simulink model "BPiKU_BAT"  (R2018b)
settings: Solver=ode23t  StartTime=0.0  StopTime=4  RelTol=1e-6
undefined symbols (not defined in the file): Cdc, i_kt_int, i_kt_p, LdM, Lout, Rd, RdM, sigbuilder_block, u_k_int, u_k_p
libraries: powerlib x29, simulink x5, powerlib_meascontrol x3
settings Model: SimulationMode=accelerator  Creator=K2  LastModifiedBy=K2

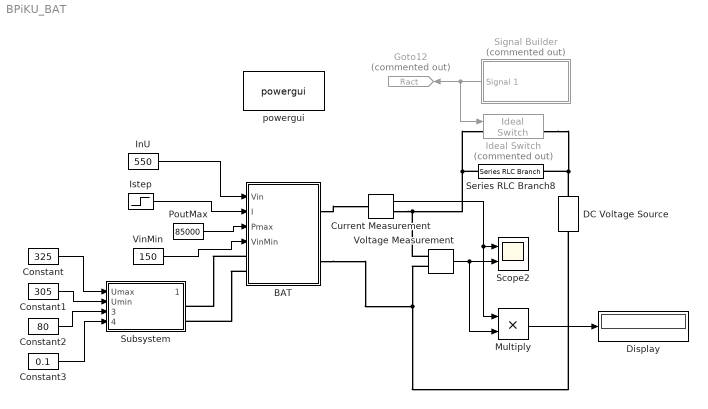
== system BPiKU_BAT ==
  BAT : Subsystem
  Constant : Constant  Value=325
  Constant1 : Constant  Value=305
  Constant2 : Constant  Value=80
  Constant3 : Constant  Value=0.1
  Current Measurement : powerlib/Measurements/Current Measurement  PhasorSimulation=off  OutputType=Complex  PSBequivalent=0
  DC Voltage Source : powerlib/Electrical Sources/DC Voltage Source  Amplitude=0  Measurements=None
  Display : Display
      settings: Format=bank
  Goto12 : Goto  Commented=on  GotoTag=Ract  TagVisibility=global
  Ideal Switch : powerlib/Power Electronics/Ideal Switch  Commented=on  Ron=550*550/85000  Lon=0  IC=0  Rs=1e5  Cs=inf  Measurements=on
  InU : Constant  Value=550
  Istep : Step  Time=0.01  After=85000/320  SampleTime=1/freq/2
  Multiply : Product
  PoutMax : Constant  Value=85000  SampleTime=0
  Scope2 : Scope  NumInputPorts=2
  Series RLC Branch8 : powerlib/Elements/Series RLC Branch  LConnTagsString=__new0  RConnTagsString=__new0  BranchType=R  Resistance=550*550/85000  Inductance=10e-6  SetiL0=off  InitialCurrent=0  Capacitance=1000e-6  Setx0=off  InitialVoltage=0  Measurements=None
  Signal Builder : Subsystem  Tag=STV Subsys  Commented=on  LoadFcn=sigbuilder_block('load');  StartFcn=sigbuilder_block('start');  StopFcn=sigbuilder_block('stop');  ClipboardFcn=sigbuilder_block('clipboard');  mask(Sigbuilder block){tuvar=[0:10]}
      mask help: Simulink:masks:SigbuilderBlock_MD
      mask init:
      | if ~strcmp(get_param(bdroot(gcbh),'SimulationStatus'),'stopped') tuvar = sigbuilder_block('maskInit'); end
      settings: CopyFcn=sigbuilder_block('copy');  DeleteFcn=sigbuilder_block('delete');  ModelCloseFcn=sigbuilder_block('modelClose');  PreSaveFcn=sigbuilder_block('preSave');  PauseFcn=sigbuilder_block('pause');  ContinueFcn=sigbuilder_block('continue');  NameChangeFcn=sigbuilder_block('namechange');  OpenFcn=sigbuilder_block('open',[193.5 84.75 550.5 399.75 ]);  CloseFcn=sigbuilder_block('close');
      mask Display: plot(0, 0, 100, 100,[2, 2, 32, 32, 2], [68, 8, 8, 68, 68],[32, 2], [38, 38], [32, 19, 2],[53, 60, 44], [32, 17, 17, 2],[16, 16, 31, 31]);txt = getActiveGroup(gcbh);text(2, 100, txt,'verticalAlignment', 'top');
  Subsystem : Subsystem
  VinMin : Constant  Value=150  SampleTime=0
  Voltage Measurement : powerlib/Measurements/Voltage Measurement  PhasorSimulation=off  OutputType=Complex  PSBequivalent=0
  powergui : powerlib/powergui  Priority=1  SimulationMode=Discrete  SampleTime=1e-6  frequency=60  Iterations=50  frequencyindice=0  Pbase=100e6  ErrMax=1e-4  UnitsV=kV  UnitsW=MW  buscounter=0  FunctionMessages=off  echomessages=off  EnableUseOfTLC=off  CurrentSourceSwitches=off  DisableSnubberDevices=off  DisableRonSwitches=off  DisableVfSwitches=off  DisplayEquations=off  SolverType=Backward Euler  Interpol=off  ExternalGateDelay=off  methode=off  Ts=100  x0status=blocks  SPID=off  SwTol=0  HookPort=off  RestoreLinks=warning  ResistiveCurrentMeasurement=off  Frange=[0:2:500]  Ylog=off  Xlog=on  ShowGrid=off  save=off  variable=ZData  structure=0  ZoomFFT=off  StartTime=0.0  cycles=1  DisplayStyle=1  fundamental=60  FreqAxis=off  MaxFrequency=1000  frequencyindicesteady=1  RmsSteady=1  display=off
  wires:
  Signal Builder/1(Signal 1) -> Ideal Switch/1, Goto12/1
  InU/1 -> BAT/1(Vin)
  Istep/1 -> BAT/2(I)
  PoutMax/1 -> BAT/3(Pmax)
  Current Measurement/1 -> Multiply/1, Scope2/1
  Voltage Measurement/1 -> Multiply/2, Scope2/2
  Multiply/1 -> Display/1
  Constant/1 -> Subsystem/1(Umax)
  Constant1/1 -> Subsystem/2(Umin)
  Constant2/1 -> Subsystem/3(InitSOC%)
  Constant3/1 -> Subsystem/4(CapMaxAh)
  VinMin/1 -> BAT/4(VinMin)
  connections:
  DC Voltage Source/RConn1 -- Ideal Switch/RConn1 -- Series RLC Branch8/RConn1
  Series RLC Branch8/LConn1 -- Voltage Measurement/LConn1 -- Current Measurement/RConn1 -- Ideal Switch/LConn1
  Voltage Measurement/LConn2 -- BAT/RConn2 -- DC Voltage Source/LConn1
  BAT/RConn1 -- Current Measurement/LConn1
  BAT/LConn1 -- Subsystem/RConn1
  BAT/LConn2 -- Subsystem/RConn2

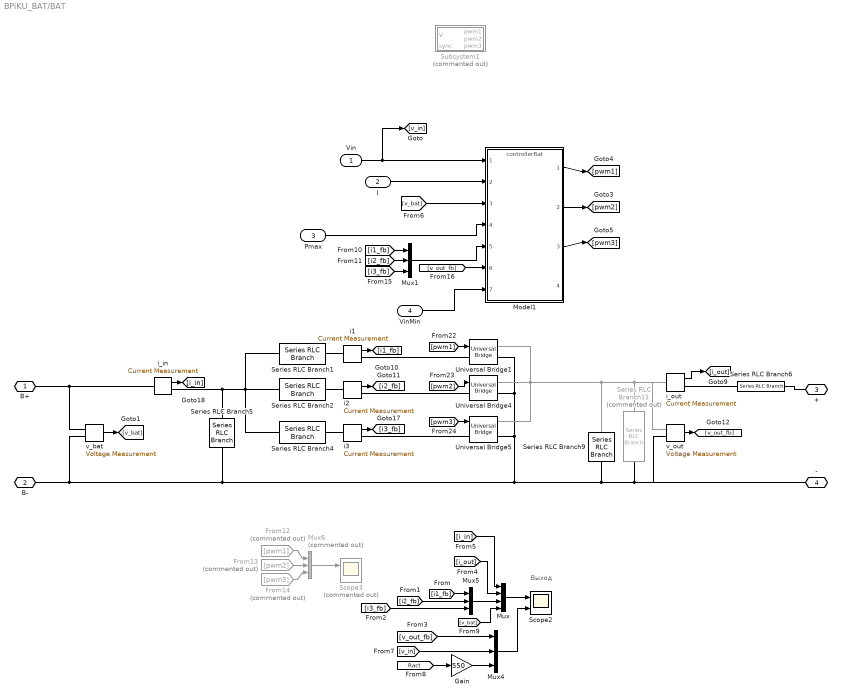
== system BPiKU_BAT/BAT ==
  note: Выход
  Vin : Inport
  I : Inport  Port=2
  Pmax : Inport  Port=3
  VinMin : Inport  Port=4
  From12 : From  Commented=on  GotoTag=pwm1
  From13 : From  Commented=on  GotoTag=pwm2
  From14 : From  Commented=on  GotoTag=pwm3
  Gain : Gain  Gain=550
  Model1 : ModelReference  ModelNameDialog=controllerBat.slx  SimulationMode=Normal  ModelReferenceVersion=1.6
  Mux : Mux
  Mux1 : Mux  Inputs=3
  Mux4 : Mux  Inputs=3
  Mux5 : Mux  Inputs=3
  Mux6 : Mux  Commented=on  Inputs=3
  Scope2 : Scope  NumInputPorts=2
  Scope3 : Scope  Commented=on  NumInputPorts=2
  Series RLC Branch1 : powerlib/Elements/Series RLC Branch  LConnTagsString=__new0  RConnTagsString=__new0  BranchType=RL  Resistance=RdM(1)  Inductance=LdM(1)  SetiL0=off  InitialCurrent=0  Capacitance=100e-6  Setx0=off  InitialVoltage=0  Measurements=None
  Series RLC Branch11 : powerlib/Elements/Series RLC Branch  Commented=on  LConnTagsString=__new0  RConnTagsString=__new0  BranchType=Open circuit  Resistance=2000  Inductance=50e-6  SetiL0=off  InitialCurrent=0  Capacitance=100e-6  Setx0=off  InitialVoltage=0  Measurements=None
  Series RLC Branch2 : powerlib/Elements/Series RLC Branch  LConnTagsString=__new0  RConnTagsString=__new0  BranchType=RL  Resistance=RdM(2)  Inductance=LdM(2)  SetiL0=off  InitialCurrent=0  Capacitance=100e-6  Setx0=off  InitialVoltage=0  Measurements=None
  Series RLC Branch4 : powerlib/Elements/Series RLC Branch  LConnTagsString=__new0  RConnTagsString=__new0  BranchType=RL  Resistance=RdM(3)  Inductance=LdM(3)  SetiL0=off  InitialCurrent=0  Capacitance=100e-6  Setx0=off  InitialVoltage=0  Measurements=None
  Series RLC Branch5 : powerlib/Elements/Series RLC Branch  LConnTagsString=__new0  RConnTagsString=__new0  BranchType=C  Resistance=0.0001  Inductance=50e-6  SetiL0=off  InitialCurrent=0  Capacitance=8000e-6  Setx0=on  InitialVoltage=300  Measurements=None
  Series RLC Branch6 : powerlib/Elements/Series RLC Branch  LConnTagsString=__new0  RConnTagsString=__new0  BranchType=RL  Resistance=Rd  Inductance=Lout  SetiL0=off  InitialCurrent=0  Capacitance=1e-6  Setx0=off  InitialVoltage=0  Measurements=None
  Series RLC Branch9 : powerlib/Elements/Series RLC Branch  LConnTagsString=__new0  RConnTagsString=__new0  BranchType=C  Resistance=0.0001  Inductance=50e-6  SetiL0=off  InitialCurrent=0  Capacitance=Cdc  Setx0=on  InitialVoltage=550  Measurements=None
  Subsystem1 : Subsystem  Commented=on
  Universal Bridge1 : powerlib/Power Electronics/Universal Bridge  Arms=1  SnubberResistance=1e5  SnubberCapacitance=inf  Device=MOSFET / Diodes  Ron=1e-3  Lon=0  ForwardVoltages="[  2  2  ]"  ForwardVoltage=0  GTOparameters=[ 10e-6 , 20e-6 ]  IGBTparameters=[ 1e-6 , 2e-6 ]  Measurements=None  Measurements_2=None  converterType=Rectifier
  Universal Bridge4 : powerlib/Power Electronics/Universal Bridge  Arms=1  SnubberResistance=1e5  SnubberCapacitance=inf  Device=MOSFET / Diodes  Ron=1e-3  Lon=0  ForwardVoltages="[  2  2  ]"  ForwardVoltage=0  GTOparameters=[ 10e-6 , 20e-6 ]  IGBTparameters=[ 1e-6 , 2e-6 ]  Measurements=None  Measurements_2=None  converterType=Rectifier
  Universal Bridge5 : powerlib/Power Electronics/Universal Bridge  Arms=1  SnubberResistance=1e5  SnubberCapacitance=inf  Device=MOSFET / Diodes  Ron=1e-3  Lon=0  ForwardVoltages="[  2  2  ]"  ForwardVoltage=0  GTOparameters=[ 10e-6 , 20e-6 ]  IGBTparameters=[ 1e-6 , 2e-6 ]  Measurements=None  Measurements_2=None  converterType=Rectifier
  i1 : powerlib/Measurements/Current Measurement  PhasorSimulation=off  OutputType=Complex  PSBequivalent=0
  i2 : powerlib/Measurements/Current Measurement  PhasorSimulation=off  OutputType=Complex  PSBequivalent=0
  i3 : powerlib/Measurements/Current Measurement  PhasorSimulation=off  OutputType=Complex  PSBequivalent=0
  i_in : powerlib/Measurements/Current Measurement  PhasorSimulation=off  OutputType=Complex  PSBequivalent=0
  i_out : powerlib/Measurements/Current Measurement  PhasorSimulation=off  OutputType=Complex  PSBequivalent=0
  v_bat : powerlib/Measurements/Voltage Measurement  PhasorSimulation=off  OutputType=Complex  PSBequivalent=0
  v_out : powerlib/Measurements/Voltage Measurement  PhasorSimulation=off  OutputType=Complex  PSBequivalent=0
  B+ : PMIOPort  Side=Left
  B- : PMIOPort  Port=2  Side=Left
  + : PMIOPort  Port=3  Side=Right
  - : PMIOPort  Port=4  Side=Right
  wires:
  From14/1 -> Mux6/3
  From12/1 -> Mux6/1
  [v_in] -> Mux4/2
  Mux5/1 -> Mux/3
  [v_out_fb] -> Mux4/1
  Mux/1 -> Scope2/1
  [i_in] -> Mux/1
  [i_out] -> Mux/2
  [i1_fb] -> Mux5/1
  From13/1 -> Mux6/2
  Mux6/1 -> Scope3/1
  [i2_fb] -> Mux5/2
  Mux4/1 -> Scope2/2
  [i3_fb] -> Mux5/3
  i3/1 -> [i3_fb]
  i1/1 -> [i1_fb]
  i2/1 -> [i2_fb]
  i_in/1 -> [i_in]
  [pwm3] -> Universal Bridge5/1
  [pwm2] -> Universal Bridge4/1
  [pwm1] -> Universal Bridge1/1
  i_out/1 -> [i_out]
  v_out/1 -> [v_out_fb]
  Model1/2 -> [pwm2]
  Model1/1 -> [pwm1]
  Vin/1 -> Model1/1, [v_in]
  Model1/3 -> [pwm3]
  I/1 -> Model1/2
  v_bat/1 -> [v_bat]
  [v_bat] -> Model1/3
  [Ract] -> Gain/1
  Gain/1 -> Mux4/3
  Pmax/1 -> Model1/4
  [v_bat] -> Mux/4
  [i2_fb] -> Mux1/2
  [i3_fb] -> Mux1/3
  [i1_fb] -> Mux1/1
  Mux1/1 -> Model1/5
  [v_out_fb] -> Model1/6
  VinMin/1 -> Model1/7
  connections:
  i_in/RConn1 -- Series RLC Branch5/LConn1 -- Series RLC Branch4/LConn1 -- Series RLC Branch2/LConn1 -- Series RLC Branch1/LConn1
  i1/LConn1 -- Series RLC Branch1/RConn1
  i3/LConn1 -- Series RLC Branch4/RConn1
  i2/RConn1 -- Universal Bridge4/LConn1
  i1/RConn1 -- Universal Bridge1/LConn1
  i2/LConn1 -- Series RLC Branch2/RConn1
  Universal Bridge5/LConn1 -- i3/RConn1
  Series RLC Branch6/RConn1 -- i_out/RConn1
  Universal Bridge5/RConn2 -- Series RLC Branch9/RConn1 -- Series RLC Branch11/RConn1 -- v_out/LConn2 -- -/RConn1 -- Series RLC Branch5/RConn1 -- v_bat/LConn2 -- B-/RConn1 -- Universal Bridge1/RConn2 -- Universal Bridge4/RConn2
  B+/RConn1 -- v_bat/LConn1 -- i_in/LConn1
  +/RConn1 -- Series RLC Branch6/LConn1
  Series RLC Branch11/LConn1 -- v_out/LConn1 -- i_out/LConn1 -- Universal Bridge5/RConn1 -- Universal Bridge1/RConn1 -- Universal Bridge4/RConn1 -- Series RLC Branch9/LConn1

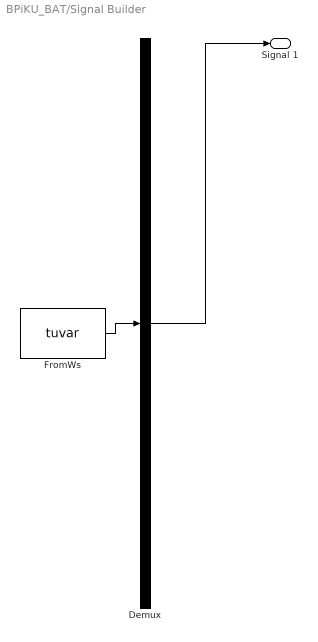
== system BPiKU_BAT/Signal Builder ==
  Demux : Demux  Tag=STV Demux  Outputs=1
  FromWs : FromWorkspace  Tag=STV FromWs  VariableName=tuvar  SampleTime=0
      SigBuilderData=|
      | common.afterFinalStr = 'Extrapolate'
      | common.sampleTime = 0
      | dataSet.timeRange = [0 10]
      | dataSet.name = 'Group 1'
      | sbobj.Groups.Name = 'Group 1'
      | sbobj.Groups.Signals.Name = 'Signal 1'
      | sbobj.Groups.Signals.XData = [0 0.02 0.51 0.51 1.5 1.5 1.88 1.88 2 2 2.07 2.07 2.15 2.15 2.24 2.24 3.58 3.58 6 10]
      | sbobj.Groups.Signals.YData = [0 0 0 1 1 0 0 1 1 0 0 1 1 0 0 1 1 0 0 0]
  Signal 1 : Outport  Tag=STV Outport
  wires:
  Demux/1 -> Signal 1/1
  FromWs/1 -> Demux/1

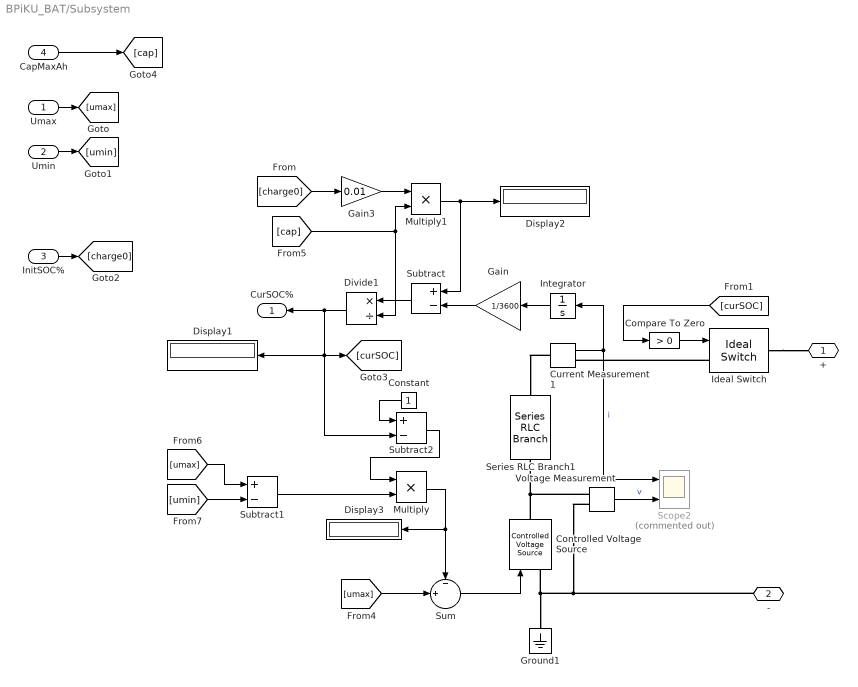
== system BPiKU_BAT/Subsystem ==
  Umax : Inport
  Umin : Inport  Port=2
  InitSOC% : Inport  Port=3
  CapMaxAh : Inport  Port=4
  Compare To Zero : simulink/Logic and Bit Operations/Compare To Zero  relop=>  OutDataTypeStr=boolean
  Constant : Constant
  Controlled Voltage Source : powerlib/Electrical Sources/Controlled Voltage Source  Initialize=on  Source_Type=AC  Amplitude=0  Phase=0  Frequency=0  Measurements=None
  Current Measurement1 : powerlib/Measurements/Current Measurement  PhasorSimulation=off  OutputType=Complex  PSBequivalent=0
  Display1 : Display
  Display2 : Display
  Display3 : Display
  Divide1 : Product  Inputs=*/
  Gain : Gain  Gain=1/3600
  Gain3 : Gain  Gain=0.01
  Ground1 : powerlib/Elements/Ground  LConnTagsString=a
  Ideal Switch : powerlib/Power Electronics/Ideal Switch  Ron=0.001  Lon=0  IC=0  Rs=1e5  Cs=inf  Measurements=off
  Integrator : Integrator
  Multiply : Product
  Multiply1 : Product
  Scope2 : Scope  Commented=on  NumInputPorts=2
  Series RLC Branch1 : powerlib/Elements/Series RLC Branch  LConnTagsString=__new0  RConnTagsString=__new0  BranchType=R  Resistance=0.01  Inductance=10e-6  SetiL0=off  InitialCurrent=0  Capacitance=1000e-6  Setx0=off  InitialVoltage=0  Measurements=None
  Subtract : Sum  Inputs=+-
  Subtract1 : Sum  Inputs=+-
  Subtract2 : Sum  Inputs=+-
  Sum : Sum  Inputs=-|+||
  Voltage Measurement : powerlib/Measurements/Voltage Measurement  PhasorSimulation=off  OutputType=Complex  PSBequivalent=0
  + : PMIOPort  Side=Right
  - : PMIOPort  Port=2  Side=Right
  CurSOC% : Outport
  wires:
  [umax] -> Sum/2
  Sum/1 -> Controlled Voltage Source/1
  Integrator/1 -> Gain/1
  Voltage Measurement/1 -> Scope2/2  "v"
  Current Measurement1/1 -> Scope2/1, Integrator/1  "i"
  Divide1/1 -> [curSOC], Subtract2/2, Display1/1, CurSOC%/1
  Umax/1 -> [umax]
  Umin/1 -> [umin]
  InitSOC%/1 -> [charge0]
  CapMaxAh/1 -> [cap]
  [charge0] -> Gain3/1
  Gain3/1 -> Multiply1/1
  [cap] -> Divide1/2, Multiply1/2
  Multiply1/1 -> Subtract/1, Display2/1
  Gain/1 -> Subtract/2
  Subtract/1 -> Divide1/1
  [umax] -> Subtract1/1
  [umin] -> Subtract1/2
  Subtract1/1 -> Multiply/2
  Multiply/1 -> Display3/1, Sum/1
  Constant/1 -> Subtract2/1
  Subtract2/1 -> Multiply/1
  [curSOC] -> Compare To Zero/1
  Compare To Zero/1 -> Ideal Switch/1
  connections:
  -/RConn1 -- Voltage Measurement/LConn2 -- Ground1/LConn1 -- Controlled Voltage Source/LConn1
  Current Measurement1/LConn1 -- Series RLC Branch1/LConn1
  Controlled Voltage Source/RConn1 -- Voltage Measurement/LConn1 -- Series RLC Branch1/RConn1
  Ideal Switch/LConn1 -- Current Measurement1/RConn1
  Ideal Switch/RConn1 -- +/RConn1

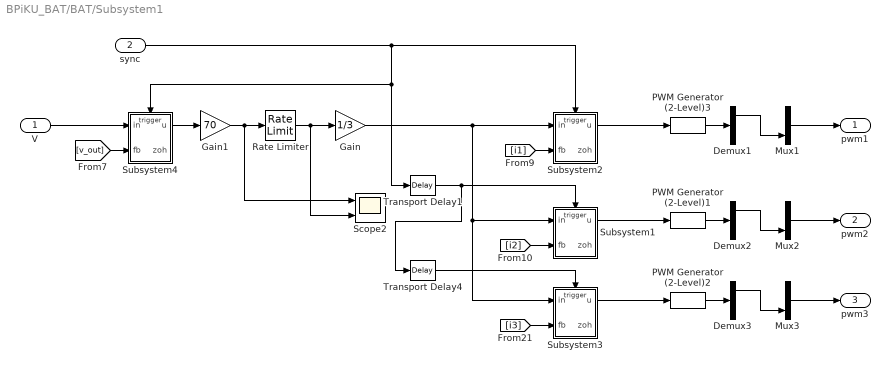
== system BPiKU_BAT/BAT/Subsystem1 ==
  V : Inport
  sync : Inport  Port=2
  Demux1 : Demux  Outputs=2
  Demux2 : Demux  Outputs=2
  Demux3 : Demux  Outputs=2
  Gain : Gain  Gain=1/3
  Gain1 : Gain  Gain=70
  Mux1 : Mux  Inputs=2
  Mux2 : Mux  Inputs=2
  Mux3 : Mux  Inputs=2
  PWM Generator (2-Level)1 : powerlib_meascontrol/Pulse & Signal Generators/PWM Generator (2-Level)  ModulatorType=Single-phase half-bridge (2 pulses)  ModulatorMode=Unsynchronized  Fc=freq  Pc=120  nF=1  MinMax="[0.001  1 ]"  SamplingTechnique=Natural  ModulatingSignals=off  m=0.8  Freq=60  Phase=0  Ts=0  ShowCarrierOutport=off
      settings: SourceProductName=Simscape Power Systems
  PWM Generator (2-Level)2 : powerlib_meascontrol/Pulse & Signal Generators/PWM Generator (2-Level)  ModulatorType=Single-phase half-bridge (2 pulses)  ModulatorMode=Unsynchronized  Fc=freq  Pc=-120  nF=1  MinMax="[0.001  1 ]"  SamplingTechnique=Natural  ModulatingSignals=off  m=0.8  Freq=60  Phase=0  Ts=0  ShowCarrierOutport=off
      settings: SourceProductName=Simscape Power Systems
  PWM Generator (2-Level)3 : powerlib_meascontrol/Pulse & Signal Generators/PWM Generator (2-Level)  ModulatorType=Single-phase half-bridge (2 pulses)  ModulatorMode=Unsynchronized  Fc=freq  Pc=0  nF=1  MinMax="[0.001  1 ]"  SamplingTechnique=Natural  ModulatingSignals=off  m=0.8  Freq=60  Phase=0  Ts=0  ShowCarrierOutport=off
      settings: SourceProductName=Simscape Power Systems
  Rate Limiter : RateLimiter  RisingSlewLimit=15  FallingSlewLimit=-15  SampleTimeMode=inherited
  Scope2 : Scope  NumInputPorts=2
  Subsystem1 : Subsystem
  Subsystem2 : Subsystem
  Subsystem3 : Subsystem
  Subsystem4 : Subsystem
  Transport Delay1 : TransportDelay  DelayTime=1/freq/2/3
  Transport Delay4 : TransportDelay  DelayTime=1/freq/2/3
  pwm1 : Outport
  pwm2 : Outport  Port=2
  pwm3 : Outport  Port=3
  wires:
  [i2] -> Subsystem1/2(fb)
  [i3] -> Subsystem3/2(fb)
  sync/1 -> Subsystem4/Trigger, Transport Delay1/1, Subsystem2/Trigger
  Transport Delay1/1 -> Subsystem1/Trigger, Transport Delay4/1
  Transport Delay4/1 -> Subsystem3/Trigger
  Mux1/1 -> pwm1/1
  Subsystem2/1(u) -> PWM Generator (2-Level)3/1
  PWM Generator (2-Level)3/1 -> Demux1/1
  Demux1/1 -> Mux1/2
  V/1 -> Subsystem4/1(in)
  [i1] -> Subsystem2/2(fb)
  Gain/1 -> Subsystem3/1(in), Subsystem1/1(in), Subsystem2/1(in)
  PWM Generator (2-Level)2/1 -> Demux3/1
  PWM Generator (2-Level)1/1 -> Demux2/1
  Mux2/1 -> pwm2/1
  [v_out] -> Subsystem4/2(fb)
  Subsystem3/1(u) -> PWM Generator (2-Level)2/1
  Demux2/1 -> Mux2/2
  Demux3/1 -> Mux3/2
  Subsystem1/1(u) -> PWM Generator (2-Level)1/1
  Subsystem4/1(u) -> Gain1/1
  Mux3/1 -> pwm3/1
  Rate Limiter/1 -> Scope2/2, Gain/1
  Gain1/1 -> Scope2/1, Rate Limiter/1

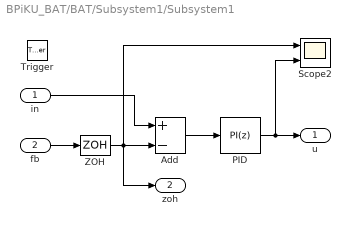
== system BPiKU_BAT/BAT/Subsystem1/Subsystem1 ==
  in : Inport
  fb : Inport  Port=2
  Trigger : TriggerPort  VariantControl=Variant  PortDimensions=1
  Add : Sum  Inputs=+-
  PID : simulink/Continuous/PID Controller  Controller=PI  Form=Parallel  TimeDomain=Discrete-time  SampleTime=-1  IntegratorMethod=Forward Euler  FilterMethod=Forward Euler  ControllerParametersSource=internal  P=i_kt_p  I=i_kt_int  D=0  UseFilter=on  N=100  TunerSelectOption=Transfer Function Based (PID Tuner App)  InitialConditionSource=internal  InitialConditionForIntegrator=0  InitialConditionForFilter=0  DifferentiatorICPrevScaledInput=0  ExternalReset=none  TrackingMode=off  Kt=1  LimitOutput=on  UpperSaturationLimit=1  LowerSaturationLimit=0  LinearizeAsGain=on  AntiWindupMode=none  Kb=1  POutMin=[]  POutMax=[]  IOutMin=[]  IOutMax=[]  DOutMin=[]  DOutMax=[]  NOutMin=[]  NOutMax=[]  SumOutMin=[]  SumOutMax=[]  SaturationOutMin=[]  SaturationOutMax=[]  PParamMin=[]  PParamMax=[]  IParamMin=[]  IParamMax=[]  DParamMin=[]  DParamMax=[]  NParamMin=[]  NParamMax=[]  KbParamMin=[]  KbParamMax=[]  KtParamMin=[]  KtParamMax=[]  KbOutMin=[]  KbOutMax=[]  KtOutMin=[]  KtOutMax=[]  IntegratorOutMin=[]  IntegratorOutMax=[]  FilterOutMin=[]  FilterOutMax=[]  SumI1OutMin=[]  SumI1OutMax=[]  SumI2OutMin=[]  SumI2OutMax=[]  SumI3OutMin=[]  SumI3OutMax=[]  SumI4OutMin=[]  SumI4OutMax=[]  SumDOutMin=[]  SumDOutMax=[]  DifferentiatorOutMin=[]  DifferentiatorOutMax=[]  FilterDiffOutCoefMin=[]  FilterDiffOutCoefMax=[]  ReciprocalOutMin=[]  ReciprocalOutMax=[]  SumDenOutMin=[]  SumDenOutMax=[]  SumNumOutMin=[]  SumNumOutMax=[]  DivideOutMin=[]  DivideOutMax=[]  IntegratorContinuousStateAttributes=''  IntegratorStateMustResolveToSignalObject=off  IntegratorRTWStateStorageClass=Auto  FilterContinuousStateAttributes=''  FilterStateMustResolveToSignalObject=off  FilterRTWStateStorageClass=Auto  ParallelPVariant=InternalParameters  IdealPVariant=Disabled  IVariant=InternalParameters  DVariant=Disabled  IntegratorVariant=Discrete  SatVariant=Enabled  AWVariant=Passthrough  PCopyVariant=Disabled  TRVariant=Disabled  FdbkBlocksVariant=Forward  IdealPFdbkVariant=Disabled  SatFdbkVariant=Disabled  DerivativeFilterVariant=Disabled  NVariant=Disabled  NCopyVariant=Disabled_SignalSpec  FilterICVariant=Disabled  IntegratorICVariant=InternalICs  ExternalResetVariant=Disabled  TRSumVariant=Passthrough  SumFdbkVariant=Disabled  SumVariant=Sum_PI
  Scope2 : Scope  NumInputPorts=2
  ZOH : ZeroOrderHold  SampleTime=-1
  u : Outport
  zoh : Outport  Port=2
  wires:
  fb/1 -> ZOH/1
  in/1 -> Add/1
  Add/1 -> PID/1
  PID/1 -> Scope2/2, u/1
  ZOH/1 -> Scope2/1, zoh/1, Add/2

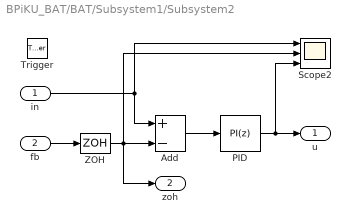
== system BPiKU_BAT/BAT/Subsystem1/Subsystem2 ==
  in : Inport
  fb : Inport  Port=2
  Trigger : TriggerPort  VariantControl=Variant  PortDimensions=1
  Add : Sum  Inputs=+-
  PID : simulink/Continuous/PID Controller  Controller=PI  Form=Parallel  TimeDomain=Discrete-time  SampleTime=-1  IntegratorMethod=Forward Euler  FilterMethod=Forward Euler  ControllerParametersSource=internal  P=i_kt_p  I=i_kt_int  D=0  UseFilter=on  N=100  TunerSelectOption=Transfer Function Based (PID Tuner App)  InitialConditionSource=internal  InitialConditionForIntegrator=0  InitialConditionForFilter=0  DifferentiatorICPrevScaledInput=0  ExternalReset=none  TrackingMode=off  Kt=1  LimitOutput=on  UpperSaturationLimit=1  LowerSaturationLimit=0  LinearizeAsGain=on  AntiWindupMode=none  Kb=1  POutMin=[]  POutMax=[]  IOutMin=[]  IOutMax=[]  DOutMin=[]  DOutMax=[]  NOutMin=[]  NOutMax=[]  SumOutMin=[]  SumOutMax=[]  SaturationOutMin=[]  SaturationOutMax=[]  PParamMin=[]  PParamMax=[]  IParamMin=[]  IParamMax=[]  DParamMin=[]  DParamMax=[]  NParamMin=[]  NParamMax=[]  KbParamMin=[]  KbParamMax=[]  KtParamMin=[]  KtParamMax=[]  KbOutMin=[]  KbOutMax=[]  KtOutMin=[]  KtOutMax=[]  IntegratorOutMin=[]  IntegratorOutMax=[]  FilterOutMin=[]  FilterOutMax=[]  SumI1OutMin=[]  SumI1OutMax=[]  SumI2OutMin=[]  SumI2OutMax=[]  SumI3OutMin=[]  SumI3OutMax=[]  SumI4OutMin=[]  SumI4OutMax=[]  SumDOutMin=[]  SumDOutMax=[]  DifferentiatorOutMin=[]  DifferentiatorOutMax=[]  FilterDiffOutCoefMin=[]  FilterDiffOutCoefMax=[]  ReciprocalOutMin=[]  ReciprocalOutMax=[]  SumDenOutMin=[]  SumDenOutMax=[]  SumNumOutMin=[]  SumNumOutMax=[]  DivideOutMin=[]  DivideOutMax=[]  IntegratorContinuousStateAttributes=''  IntegratorStateMustResolveToSignalObject=off  IntegratorRTWStateStorageClass=Auto  FilterContinuousStateAttributes=''  FilterStateMustResolveToSignalObject=off  FilterRTWStateStorageClass=Auto  ParallelPVariant=InternalParameters  IdealPVariant=Disabled  IVariant=InternalParameters  DVariant=Disabled  IntegratorVariant=Discrete  SatVariant=Enabled  AWVariant=Passthrough  PCopyVariant=Disabled  TRVariant=Disabled  FdbkBlocksVariant=Forward  IdealPFdbkVariant=Disabled  SatFdbkVariant=Disabled  DerivativeFilterVariant=Disabled  NVariant=Disabled  NCopyVariant=Disabled_SignalSpec  FilterICVariant=Disabled  IntegratorICVariant=InternalICs  ExternalResetVariant=Disabled  TRSumVariant=Passthrough  SumFdbkVariant=Disabled  SumVariant=Sum_PI
  Scope2 : Scope  NumInputPorts=3
  ZOH : ZeroOrderHold  SampleTime=-1
  u : Outport
  zoh : Outport  Port=2
  wires:
  fb/1 -> ZOH/1
  in/1 -> Scope2/1, Add/1
  Add/1 -> PID/1
  PID/1 -> Scope2/3, u/1
  ZOH/1 -> Scope2/2, zoh/1, Add/2

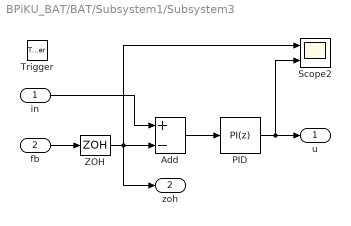
== system BPiKU_BAT/BAT/Subsystem1/Subsystem3 ==
  in : Inport
  fb : Inport  Port=2
  Trigger : TriggerPort  VariantControl=Variant  PortDimensions=1
  Add : Sum  Inputs=+-
  PID : simulink/Continuous/PID Controller  Controller=PI  Form=Parallel  TimeDomain=Discrete-time  SampleTime=-1  IntegratorMethod=Forward Euler  FilterMethod=Forward Euler  ControllerParametersSource=internal  P=i_kt_p  I=i_kt_int  D=0  UseFilter=on  N=100  TunerSelectOption=Transfer Function Based (PID Tuner App)  InitialConditionSource=internal  InitialConditionForIntegrator=0  InitialConditionForFilter=0  DifferentiatorICPrevScaledInput=0  ExternalReset=none  TrackingMode=off  Kt=1  LimitOutput=on  UpperSaturationLimit=1  LowerSaturationLimit=0  LinearizeAsGain=on  AntiWindupMode=none  Kb=1  POutMin=[]  POutMax=[]  IOutMin=[]  IOutMax=[]  DOutMin=[]  DOutMax=[]  NOutMin=[]  NOutMax=[]  SumOutMin=[]  SumOutMax=[]  SaturationOutMin=[]  SaturationOutMax=[]  PParamMin=[]  PParamMax=[]  IParamMin=[]  IParamMax=[]  DParamMin=[]  DParamMax=[]  NParamMin=[]  NParamMax=[]  KbParamMin=[]  KbParamMax=[]  KtParamMin=[]  KtParamMax=[]  KbOutMin=[]  KbOutMax=[]  KtOutMin=[]  KtOutMax=[]  IntegratorOutMin=[]  IntegratorOutMax=[]  FilterOutMin=[]  FilterOutMax=[]  SumI1OutMin=[]  SumI1OutMax=[]  SumI2OutMin=[]  SumI2OutMax=[]  SumI3OutMin=[]  SumI3OutMax=[]  SumI4OutMin=[]  SumI4OutMax=[]  SumDOutMin=[]  SumDOutMax=[]  DifferentiatorOutMin=[]  DifferentiatorOutMax=[]  FilterDiffOutCoefMin=[]  FilterDiffOutCoefMax=[]  ReciprocalOutMin=[]  ReciprocalOutMax=[]  SumDenOutMin=[]  SumDenOutMax=[]  SumNumOutMin=[]  SumNumOutMax=[]  DivideOutMin=[]  DivideOutMax=[]  IntegratorContinuousStateAttributes=''  IntegratorStateMustResolveToSignalObject=off  IntegratorRTWStateStorageClass=Auto  FilterContinuousStateAttributes=''  FilterStateMustResolveToSignalObject=off  FilterRTWStateStorageClass=Auto  ParallelPVariant=InternalParameters  IdealPVariant=Disabled  IVariant=InternalParameters  DVariant=Disabled  IntegratorVariant=Discrete  SatVariant=Enabled  AWVariant=Passthrough  PCopyVariant=Disabled  TRVariant=Disabled  FdbkBlocksVariant=Forward  IdealPFdbkVariant=Disabled  SatFdbkVariant=Disabled  DerivativeFilterVariant=Disabled  NVariant=Disabled  NCopyVariant=Disabled_SignalSpec  FilterICVariant=Disabled  IntegratorICVariant=InternalICs  ExternalResetVariant=Disabled  TRSumVariant=Passthrough  SumFdbkVariant=Disabled  SumVariant=Sum_PI
  Scope2 : Scope  NumInputPorts=2
  ZOH : ZeroOrderHold  SampleTime=-1
  u : Outport
  zoh : Outport  Port=2
  wires:
  fb/1 -> ZOH/1
  in/1 -> Add/1
  Add/1 -> PID/1
  PID/1 -> Scope2/2, u/1
  ZOH/1 -> Scope2/1, zoh/1, Add/2

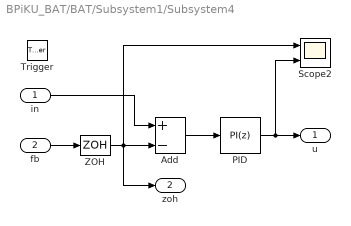
== system BPiKU_BAT/BAT/Subsystem1/Subsystem4 ==
  in : Inport
  fb : Inport  Port=2
  Trigger : TriggerPort  VariantControl=Variant  PortDimensions=1
  Add : Sum  Inputs=+-
  PID : simulink/Continuous/PID Controller  Controller=PI  Form=Parallel  TimeDomain=Discrete-time  SampleTime=-1  IntegratorMethod=Forward Euler  FilterMethod=Forward Euler  ControllerParametersSource=internal  P=u_k_p  I=u_k_int  D=0  UseFilter=on  N=100  TunerSelectOption=Transfer Function Based (PID Tuner App)  InitialConditionSource=internal  InitialConditionForIntegrator=0  InitialConditionForFilter=0  DifferentiatorICPrevScaledInput=0  ExternalReset=none  TrackingMode=off  Kt=1  LimitOutput=on  UpperSaturationLimit=1  LowerSaturationLimit=0  LinearizeAsGain=on  AntiWindupMode=none  Kb=1  POutMin=[]  POutMax=[]  IOutMin=[]  IOutMax=[]  DOutMin=[]  DOutMax=[]  NOutMin=[]  NOutMax=[]  SumOutMin=[]  SumOutMax=[]  SaturationOutMin=[]  SaturationOutMax=[]  PParamMin=[]  PParamMax=[]  IParamMin=[]  IParamMax=[]  DParamMin=[]  DParamMax=[]  NParamMin=[]  NParamMax=[]  KbParamMin=[]  KbParamMax=[]  KtParamMin=[]  KtParamMax=[]  KbOutMin=[]  KbOutMax=[]  KtOutMin=[]  KtOutMax=[]  IntegratorOutMin=[]  IntegratorOutMax=[]  FilterOutMin=[]  FilterOutMax=[]  SumI1OutMin=[]  SumI1OutMax=[]  SumI2OutMin=[]  SumI2OutMax=[]  SumI3OutMin=[]  SumI3OutMax=[]  SumI4OutMin=[]  SumI4OutMax=[]  SumDOutMin=[]  SumDOutMax=[]  DifferentiatorOutMin=[]  DifferentiatorOutMax=[]  FilterDiffOutCoefMin=[]  FilterDiffOutCoefMax=[]  ReciprocalOutMin=[]  ReciprocalOutMax=[]  SumDenOutMin=[]  SumDenOutMax=[]  SumNumOutMin=[]  SumNumOutMax=[]  DivideOutMin=[]  DivideOutMax=[]  IntegratorContinuousStateAttributes=''  IntegratorStateMustResolveToSignalObject=off  IntegratorRTWStateStorageClass=Auto  FilterContinuousStateAttributes=''  FilterStateMustResolveToSignalObject=off  FilterRTWStateStorageClass=Auto  ParallelPVariant=InternalParameters  IdealPVariant=Disabled  IVariant=InternalParameters  DVariant=Disabled  IntegratorVariant=Discrete  SatVariant=Enabled  AWVariant=Passthrough  PCopyVariant=Disabled  TRVariant=Disabled  FdbkBlocksVariant=Forward  IdealPFdbkVariant=Disabled  SatFdbkVariant=Disabled  DerivativeFilterVariant=Disabled  NVariant=Disabled  NCopyVariant=Disabled_SignalSpec  FilterICVariant=Disabled  IntegratorICVariant=InternalICs  ExternalResetVariant=Disabled  TRSumVariant=Passthrough  SumFdbkVariant=Disabled  SumVariant=Sum_PI
  Scope2 : Scope  NumInputPorts=2
  ZOH : ZeroOrderHold  SampleTime=-1
  u : Outport
  zoh : Outport  Port=2
  wires:
  fb/1 -> ZOH/1
  in/1 -> Add/1
  Add/1 -> PID/1
  PID/1 -> Scope2/2, u/1
  ZOH/1 -> Scope2/1, zoh/1, Add/2
